simulink model "EngineCtrl_MILS"  (R2018a)
settings: Solver=ode23s  StartTime=0.0  StopTime=10.0  RelTol=1e-3
settings Model: Creator=nishito  LastModifiedBy=nishito
settings CodeAppCC: StateflowObjectComments=on

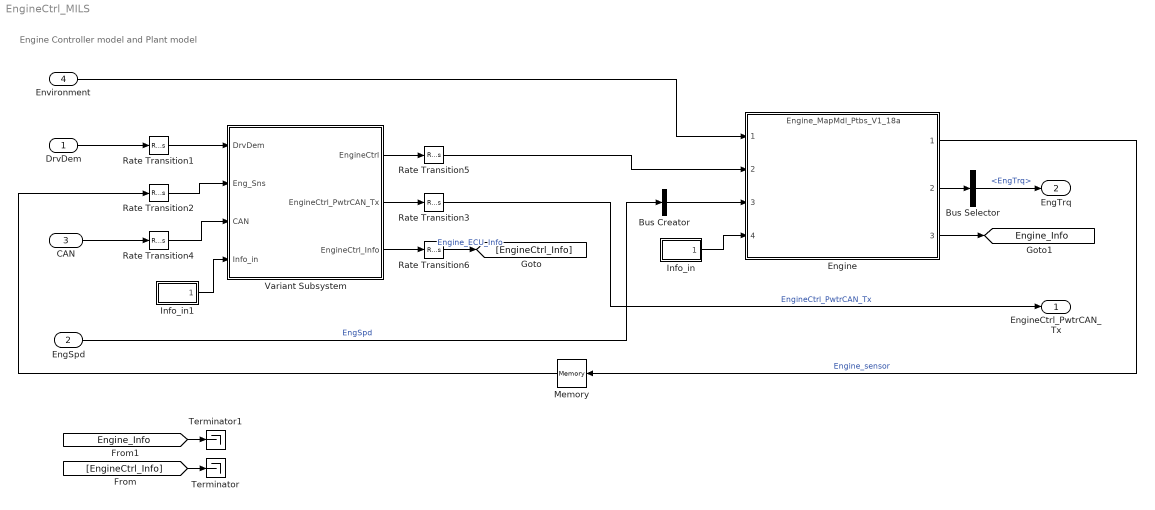
== system EngineCtrl_MILS ==
  note: Engine Controller model and Plant model
  DrvDem : Inport  OutDataTypeStr=Bus: Driver_demand_Bus
      settings: AttributesFormatString=%<OutDataTypeStr>
  EngSpd : Inport  Port=2
  CAN : Inport  Port=3  OutDataTypeStr=Bus: CAN_Bus
      settings: AttributesFormatString=%<OutDataTypeStr>
  Environment : Inport  Port=4  OutDataTypeStr=Bus: Environment_Bus
      settings: AttributesFormatString=%<OutDataTypeStr>
  Bus Creator : BusCreator  Inputs=1
  Bus Selector : BusSelector  OutputSignals=EngTrq
  Engine : ModelReference  ModelNameDialog=Engine_MapMdl_Ptbs_V1_18a.slx  SimulationMode=Normal  ModelReferenceVersion=1.1337
  Info_in : Subsystem
  Info_in1 : Subsystem
  Memory : Memory
  Rate Transition{1..6} (6 alike) : RateTransition  Deterministic=off
      settings: AttributesFormatString=<Deterministic=%<Deterministic>>
  Terminator : Terminator
  Terminator1 : Terminator
  Variant Subsystem : Subsystem  Variant=on  OverrideUsingVariant=Variant
  EngineCtrl_PwtrCAN_Tx : Outport
  EngTrq : Outport  Port=2
  tag scope: Engine_Info=global
  wires:
  DrvDem/1 -> Rate Transition1/1
  Variant Subsystem/3(EngineCtrl_Info) -> Rate Transition6/1
  CAN/1 -> Rate Transition4/1
  Variant Subsystem/1(EngineCtrl) -> Rate Transition5/1
  Rate Transition1/1 -> Variant Subsystem/1(DrvDem)
  Rate Transition4/1 -> Variant Subsystem/3(CAN)
  Variant Subsystem/2(EngineCtrl_PwtrCAN_Tx) -> Rate Transition3/1
  Rate Transition6/1 -> [EngineCtrl_Info]  "Engine_ECU_Info"
  Rate Transition3/1 -> EngineCtrl_PwtrCAN_Tx/1  "EngineCtrl_PwtrCAN_Tx"
  Rate Transition2/1 -> Variant Subsystem/2(Eng_Sns)
  [EngineCtrl_Info] -> Terminator/1
  [Engine_Info] -> Terminator1/1
  Engine/3 -> [Engine_Info]
  Engine/1 -> Memory/1  "Engine_sensor"
  Environment/1 -> Engine/1
  Bus Selector/1 -> EngTrq/1  "<EngTrq>"
  Info_in/1(Info_in) -> Engine/4
  Rate Transition5/1 -> Engine/2
  Bus Creator/1 -> Engine/3
  EngSpd/1 -> Bus Creator/1  "EngSpd"
  Memory/1 -> Rate Transition2/1
  Info_in1/1(Info_in) -> Variant Subsystem/4(Info_in)
  Engine/2 -> Bus Selector/1

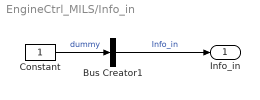
== system EngineCtrl_MILS/Info_in ==
  Bus Creator1 : BusCreator  Inputs=1
  Constant : Constant
  Info_in : Outport
  wires:
  Constant/1 -> Bus Creator1/1  "dummy"
  Bus Creator1/1 -> Info_in/1  "Info_in"

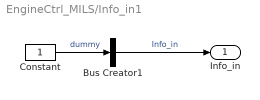
== system EngineCtrl_MILS/Info_in1 ==
  Bus Creator1 : BusCreator  Inputs=1
  Constant : Constant
  Info_in : Outport
  wires:
  Bus Creator1/1 -> Info_in/1  "Info_in"
  Constant/1 -> Bus Creator1/1  "dummy"

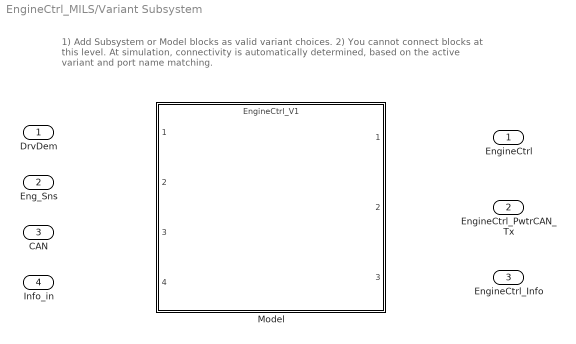
== system EngineCtrl_MILS/Variant Subsystem ==
  note: 1) Add Subsystem or Model blocks as valid variant choices.
      | 2) You cannot connect blocks at this level. At simulation, connectivity is automatically
      | determined, based on the active variant and port name matching.
  DrvDem : Inport
  Eng_Sns : Inport  Port=2
  CAN : Inport  Port=3
  Info_in : Inport  Port=4
  Model : ModelReference  ModelNameDialog=EngineCtrl_V1.slx  SimulationMode=Normal  VariantControl=Variant  ModelReferenceVersion=1.0.18
  EngineCtrl : Outport
  EngineCtrl_PwtrCAN_Tx : Outport  Port=2
  EngineCtrl_Info : Outport  Port=3
